simulink model "StateSpaceSim"  (R2020b)
settings: Solver=ode45  StartTime=0.0  StopTime=10  FixedStep=1ms  RelTol=1e-3
undefined symbols (not defined in the file or in its folder): daq, degs2rpm, drv, gbox, mech, mld, mot, rads2rpm, rpm2rads, sens, ss
libraries: simulink x1
settings Model: Creator=Utente  LastModifiedBy=Utente

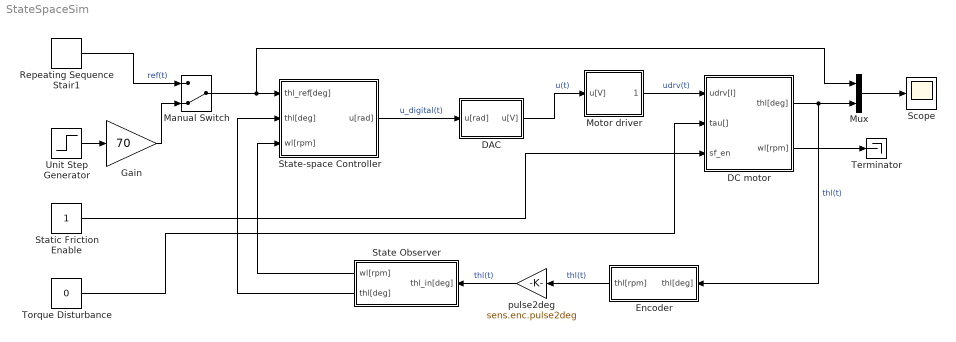
== system StateSpaceSim ==
  DAC : Subsystem
  DC motor : Subsystem
  Encoder : Subsystem
  Gain : Gain  Gain=70
  Manual Switch : ManualSwitch  CurrentSetting=0
  Motor driver : Subsystem
  Mux : Mux  Inputs=2
  Repeating Sequence Stair1 : simulink/Sources/Repeating Sequence Stair  OutValues=[40 0 70 0 120 0].'  tsamp=2  OutMin=[]  OutMax=[]  OutDataTypeStr=double  OutputDataTypeScalingMode=double  OutDataType=fixdt(0,8)  ConRadixGroup=Best Precision: Vector-wise  OutScaling=2^-12
  Scope : Scope
  State Observer : Subsystem
  State-space Controller : Subsystem
  Static Friction Enable : Constant
  Terminator : Terminator
  Torque Disturbance : Constant  Value=0
  Unit Step Generator : Step  Time=0  SampleTime=0
  pulse2deg : Gain  Gain=sens.enc.pulse2deg
  wires:
  pulse2deg/1 -> State Observer/1(thl_in[deg])  "thl(t)"
  Encoder/1(thl[rpm]) -> pulse2deg/1  "thl(t)"
  DAC/1(u[V]) -> Motor driver/1(u[V])  "u(t)"
  State-space Controller/1(u[rad]) -> DAC/1(u[rad])  "u_digital(t)"
  State Observer/1(wl[rpm]) -> State-space Controller/3(wl[rpm])
  State Observer/2(thl[deg]) -> State-space Controller/2(thl[deg])
  DC motor/1(thl[deg]) -> Mux/2, Encoder/1(thl[deg])  "thl(t)"
  Mux/1 -> Scope/1
  Manual Switch/1 -> Mux/1, State-space Controller/1(thl_ref[deg])
  Motor driver/1(udrv[I]) -> DC motor/1(udrv[I])  "udrv(t)"
  DC motor/2(wl[rpm]) -> Terminator/1
  Torque Disturbance/1 -> DC motor/2(tau[])
  Static Friction Enable/1 -> DC motor/3(sf_en)
  Unit Step Generator/1 -> Gain/1
  Repeating Sequence Stair1/1 -> Manual Switch/1  "ref(t)"
  Gain/1 -> Manual Switch/2

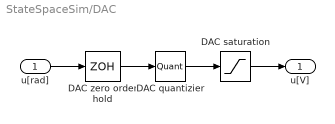
== system StateSpaceSim/DAC ==
  u[rad] : Inport
  DAC quantizier : Quantizer  QuantizationInterval=daq.dac.q
  DAC saturation : Saturate  UpperLimit=daq.dac.vdd  LowerLimit=daq.dac.vss
  DAC zero order hold : ZeroOrderHold  SampleTime=daq.dac.T_s
  u[V] : Outport
  wires:
  DAC quantizier/1 -> DAC saturation/1
  DAC zero order hold/1 -> DAC quantizier/1
  DAC saturation/1 -> u[V]/1
  u[rad]/1 -> DAC zero order hold/1

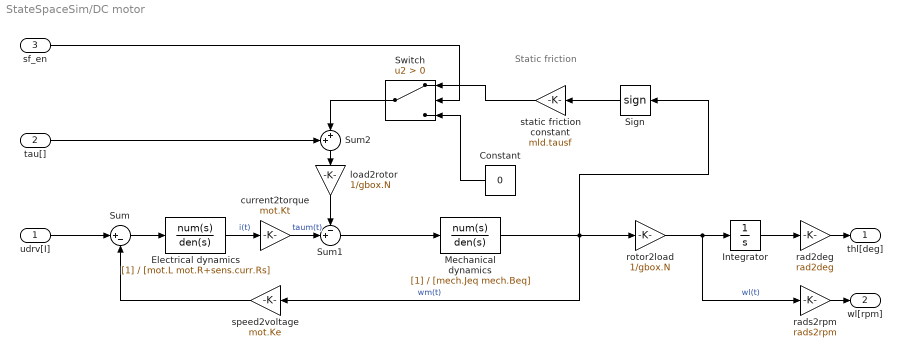
== system StateSpaceSim/DC motor ==
  note: Static friction
  udrv[I] : Inport  Unit=V
  tau[] : Inport  Port=2  Unit=V
  sf_en : Inport  Port=3  Unit=V
  Constant : Constant  Value=0
  Electrical dynamics : TransferFcn  Denominator=[mot.L mot.R+sens.curr.Rs]
  Integrator : Integrator
  Mechanical dynamics : TransferFcn  Denominator=[mech.Jeq mech.Beq]
  Sign : Signum  ZeroCross=off
  Sum : Sum  Inputs=|+-
  Sum1 : Sum  Inputs=-+|
  Sum2 : Sum  Inputs=++|
  Switch : Switch  Criteria=u2 > Threshold
  current2torque : Gain  Gain=mot.Kt
  load2rotor : Gain  Gain=1/gbox.N
  rad2deg : Gain  Gain=rad2deg
  rads2rpm : Gain  Gain=rads2rpm
  rotor2load : Gain  Gain=1/gbox.N
  speed2voltage : Gain  Gain=mot.Ke
  static friction constant : Gain  Gain=mld.tausf
  thl[deg] : Outport  Unit=deg
  wl[rpm] : Outport  Port=2  Unit=rpm
  wires:
  load2rotor/1 -> Sum1/1
  Mechanical dynamics/1 -> Sign/1, rotor2load/1, speed2voltage/1  "wm(t)"
  Sign/1 -> static friction constant/1
  current2torque/1 -> Sum1/2  "taum(t)"
  Sum1/1 -> Mechanical dynamics/1
  speed2voltage/1 -> Sum/2
  rotor2load/1 -> rads2rpm/1, Integrator/1  "wl(t)"
  Electrical dynamics/1 -> current2torque/1  "i(t)"
  Integrator/1 -> rad2deg/1
  Sum/1 -> Electrical dynamics/1
  rads2rpm/1 -> wl[rpm]/1
  rad2deg/1 -> thl[deg]/1
  udrv[I]/1 -> Sum/1
  Sum2/1 -> load2rotor/1
  tau[]/1 -> Sum2/1
  Switch/1 -> Sum2/2
  static friction constant/1 -> Switch/1
  Constant/1 -> Switch/3
  sf_en/1 -> Switch/2

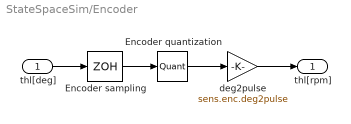
== system StateSpaceSim/Encoder ==
  thl[deg] : Inport
  Encoder quantization : Quantizer  QuantizationInterval=sens.enc.q
  Encoder sampling : ZeroOrderHold  SampleTime=sens.enc.T_s
  deg2pulse : Gain  Gain=sens.enc.deg2pulse
  thl[rpm] : Outport
  wires:
  Encoder quantization/1 -> deg2pulse/1
  deg2pulse/1 -> thl[rpm]/1
  Encoder sampling/1 -> Encoder quantization/1
  thl[deg]/1 -> Encoder sampling/1

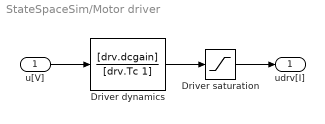
== system StateSpaceSim/Motor driver ==
  u[V] : Inport
  Driver dynamics : TransferFcn  Numerator=[drv.dcgain]  Denominator=[drv.Tc 1]
  Driver saturation : Saturate  UpperLimit=drv.vp  LowerLimit=drv.vm
  udrv[I] : Outport
  wires:
  Driver saturation/1 -> udrv[I]/1
  Driver dynamics/1 -> Driver saturation/1
  u[V]/1 -> Driver dynamics/1

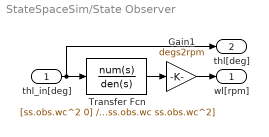
== system StateSpaceSim/State Observer ==
  thl_in[deg] : Inport
  Gain1 : Gain  Gain=degs2rpm
  Transfer Fcn : TransferFcn  Numerator=[ss.obs.wc^2 0]  Denominator=[1 2*ss.obs.delta*ss.obs.wc ss.obs.wc^2]
  wl[rpm] : Outport
  thl[deg] : Outport  Port=2
  wires:
  Transfer Fcn/1 -> Gain1/1
  thl_in[deg]/1 -> thl[deg]/1, Transfer Fcn/1
  Gain1/1 -> wl[rpm]/1

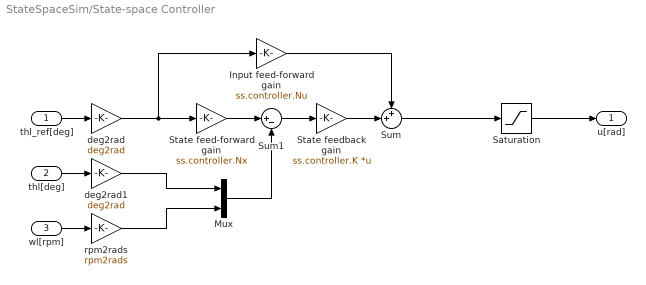
== system StateSpaceSim/State-space Controller ==
  thl_ref[deg] : Inport
  thl[deg] : Inport  Port=2
  wl[rpm] : Inport  Port=3
  Input feed-forward gain : Gain  Gain=ss.controller.Nu
  Mux : Mux  Inputs=2
  Saturation : Saturate  UpperLimit=daq.dac.vdd  LowerLimit=daq.dac.vss
  State feed-forward gain : Gain  Gain=ss.controller.Nx
  State feedback gain : Gain  Gain=ss.controller.K  Multiplication=Matrix(K*u)
  Sum : Sum  Inputs=++|
  Sum1 : Sum  Inputs=|+-
  deg2rad : Gain  Gain=deg2rad
  deg2rad1 : Gain  Gain=deg2rad
  rpm2rads : Gain  Gain=rpm2rads
  u[rad] : Outport
  wires:
  rpm2rads/1 -> Mux/2
  Sum1/1 -> State feedback gain/1
  Mux/1 -> Sum1/2
  thl_ref[deg]/1 -> deg2rad/1
  deg2rad/1 -> Input feed-forward gain/1, State feed-forward gain/1
  State feed-forward gain/1 -> Sum1/1
  deg2rad1/1 -> Mux/1
  Input feed-forward gain/1 -> Sum/1
  Saturation/1 -> u[rad]/1
  wl[rpm]/1 -> rpm2rads/1
  thl[deg]/1 -> deg2rad1/1
  State feedback gain/1 -> Sum/2
  Sum/1 -> Saturation/1
